simulink model "GDFLIB_FilterIIR1_BAM"  (Simulink 9.3)
settings: Solver=VariableStepAuto  StartTime=0.0  StopTime=10.0  RelTol=1e-3
settings Model: Creator=nxa18952  LastModifiedBy=nxa18952
settings DataIOCC: SaveFormat=Dataset  SignalLoggingSaveFormat=Dataset  ReturnWorkspaceOutputs=on
settings OptimizationCC: LifeSpan=auto
settings DebuggingCC: UnderspecifiedInitializationDetection=Simplified  MergeDetectMultiDrivingBlocksExec=error  FcnCallInpInsideContextMsg=error  SFUnexpectedBacktrackingDiag=error  SFNoUnconditionalDefaultTransitionDiag=error  SFExecutionAtInitializationDiag=warning  ArithmeticOperatorsInVariantConditions=error
settings HardwareCC: ProdBitPerPointer=64  ProdBitPerSizeT=64  ProdBitPerPtrDiffT=64  ProdLargestAtomicFloat=Float  ProdIntDivRoundTo=Zero  ProdEndianess=LittleEndian  ProdWordSize=64  ProdHWDeviceType=Intel->x86-64 (Windows64)
settings ModelReferenceCC: PropagateSignalLabelsOutOfModel=on
settings SFSimCC: SimUseLocalCustomCode=on
settings RTWCC: RTWUseLocalCustomCode=on
settings CodeAppCC: StateflowObjectComments=off
settings GRTTargetCC: TargetLangStandard=C99 (ISO)  CombineOutputUpdateFcns=on  GRTInterface=off
settings ConfigComp: CovMetricSettings=dwe  CovHtmlReporting=off  CovSaveCumulativeToWorkspaceVar=off  CovSaveSingleToWorkspaceVar=off  CovExternalEMLEnable=on

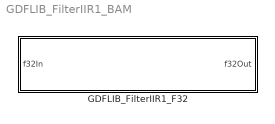
== system GDFLIB_FilterIIR1_BAM ==
  GDFLIB_FilterIIR1_F32 : Subsystem  TreatAsAtomicUnit=on  mask(GDFLIB_FilterIIR1_F32){showStates=Hide (faster execution), f32B0=0, f32B1=0, f32A1=0}
      mask prompts: showStates "Show internal states"; f32B0 "f32B0 (B0 coefficient of the IIR1 filter in 32-bit fixed-point fractional format)"; f32B1 "f32B1 (B1 coefficient of the IIR1 filter in 32-bit fixed-point fractional format)"; f32A1 "f32A1 (A1 coefficient of the IIR1 filter in 32-bit fixed-point fractional format)"
      mask help: Direct form I first order IIR filter in 32-bit fixed-point fractional implementation. Refer to the AMMCLIB User's Guide for further details.
      mask init:
      | if ~evalin('base','exist(''tS8'',''var'')')
      |   if (2 ~= exist('SWLIBS_Typedefs.mat','file'))
      |       error('File SWLIBS_Typedefs.mat is not on the Matlab path. Please add the AMMCLIB "bam" folder in the Matlab Search Path.');
      |   else
      |       evalin('base', 'load(''SWLIBS_Typedefs.mat'')');
      |   end
      | end
      | if showStates == 1
      |     % hidden state variables
      |     if strcmp(get_param([gcb '/f32B0'], 'BlockType'), 'Inport')
      |         posblk = get_param(gcb, 'Position');
      | 
      |         pos = get_param(    [gcb, '/f32B0'], 'Position');
      |         orient = get_param( [gcb, '/f32B0'], 'Orientation');
      |         delete_block(       [gcb, '/f32B0']);
      |         add_block('built-in/Ground', [gcb, '/f32B0'], 'Position', pos, 'Orientation', orient);
      | 
      |         pos = get_param(    [gcb, '/f32B1'], 'Position');
      |         orient = get_param( [gcb, '/f32B1'], 'Orientation');
      |         delete_block(       [gcb, '/f32B1']);
      |         add_block('built-in/Ground', [gcb, '/f32B1'], 'Position', pos, 'Orientation', orient);
      | 
      |         pos = get_param(    [gcb, '/f32A1'], 'Position');
      |         orient = get_param( [gcb, '/f32A1'], 'Orientation');
      |         delete_block(       [gcb, '/f32A1']);
      |         add_block('built-in/Ground', [gcb, '/f32A1'], 'Position', pos, 'Orientation', orient);
      | 
      |         pos = get_param(    [gcb, '/f32FiltBufferX'], 'Position');
      |         orient = get_param( [gcb, '/f32FiltBufferX'], 'Orientation');
      |         delete_block(       [gcb, '/f32FiltBufferX']);
      |         add_block('built-in/Ground', [gcb, '/f32FiltBufferX'], 'Position', pos, 'Orientation', orient);
      | 
      |         pos = get_param(    [gcb, '/f32FiltBufferY'], 'Position');
      |         orient = get_param( [gcb, '/f32FiltBufferY'], 'Orientation');
      |         delete_block(       [gcb, '/f32FiltBufferY']);
      |         add_block('built-in/Ground', [gcb, '/f32FiltBufferY'], 'Position', pos, 'Orientation', orient);
      | 
      | 
      |         pos = get_param(    [gcb '/f32FiltBufferX_Out'], 'Position');
      |         orient = get_param( [gcb '/f32FiltBufferX_Out'], 'Orientation');
      |         delete_block(       [gcb '/f32FiltBufferX_Out']);
      |         add_block('built-in/Terminator', [gcb '/f32FiltBufferX_Out'], 'Position', pos, 'Orientation', orient);
      | 
      |         pos = get_param(    [gcb '/f32FiltBufferY_Out'], 'Position');
      |         orient = get_param( [gcb '/f32FiltBufferY_Out'], 'Orientation');
      |         delete_block(       [gcb '/f32FiltBufferY_Out']);
      |         add_block('built-in/Terminator', [gcb '/f32FiltBufferY_Out'], 'Position', pos, 'Orientation', orient);
      | 
      | 
      |         set_param([gcb '/f32In'], 'Port', '1');
      | 
      |         set_param([gcb '/f32Out'], 'Port', '1');
      | 
      |         set_param(gcb,'MaskEnables',{'on','on','on','on'});
      | 
      |         if (posblk(4) - posblk(2)) > 50
      |           height = 50;
      |           set_param(gcb,'Position',[posblk(1), posblk(2), posblk(3), posblk(2)+height])
      |         end
      |     end
      | else
      |     % shown state variables
      |     if strcmp(get_param([gcb '/f32B0'], 'BlockType'), 'Ground')
      |         posblk = get_param(gcb, 'Position');
      | 
      |         pos = get_param(    [gcb, '/f32B0'], 'Position');
      |         orient = get_param( [gcb, '/f32B0'], 'Orientation');
      |         delete_block(       [gcb, '/f32B0']);
      |         add_block('built-in/Inport', [gcb, '/f32B0'], 'Position', pos, 'Orientation', orient, 'OutDataTypeStr', 'int32');
      | 
      |         pos = get_param(    [gcb, '/f32B1'], 'Position');
      |         orient = get_param( [gcb, '/f32B1'], 'Orientation');
      |         delete_block(       [gcb, '/f32B1']);
      |         add_block('built-in/Inport', [gcb, '/f32B1'], 'Position', pos, 'Orientation', orient, 'OutDataTypeStr', 'int32');
      | 
      |         pos = get_param(    [gcb, '/f32A1'], 'Position');
      |         orient = get_param( [gcb, '/f32A1'], 'Orientation');
      |         delete_block(       [gcb, '/f32A1']);
      |         add_block('built-in/Inport', [gcb, '/f32A1'], 'Position', pos, 'Orientation', orient, 'OutDataTypeStr', 'int32');
      | 
      |         pos = get_param(    [gcb, '/f32FiltBufferX'], 'Position');
      |         orient = get_param( [gcb, '/f32FiltBufferX'], 'Orientation');
      |         delete_block(       [gcb, '/f32FiltBufferX']);
      |         add_block('built-in/Inport', [gcb, '/f32FiltBufferX'], 'Position', pos, 'Orientation', orient, 'OutDataTypeStr', 'int32');
      | 
      |         pos = get_param(    [gcb, '/f32FiltBufferY'], 'Position');
      |         orient = get_param( [gcb, '/f32FiltBufferY'], 'Orientation');
      |         delete_block(       [gcb, '/f32FiltBufferY']);
      |         add_block('built-in/Inport', [gcb, '/f32FiltBufferY'], 'Position', pos, 'Orientation', orient, 'OutDataTypeStr', 'int32');
      | 
      | 
      |         pos = get_param(    [gcb '/f32FiltBufferX_Out'], 'Position');
      |         orient = get_param( [gcb '/f32FiltBufferX_Out'], 'Orientation');
      |         delete_block(       [gcb '/f32FiltBufferX_Out']);
      |         add_block('built-in/Outport', [gcb '/f32FiltBufferX_Out'], 'Position', pos, 'Orientation', orient);
      | 
      |         pos = get_param(    [gcb '/f32FiltBufferY_Out'], 'Position');
      |         orient = get_param( [gcb '/f32FiltBufferY_Out'], 'Orientation');
      |         delete_block(       [gcb '/f32FiltBufferY_Out']);
      |         add_block('built-in/Outport', [gcb '/f32FiltBufferY_Out'], 'Position', pos, 'Orientation', orient);
      | 
      | 
      |         set_param([gcb '/f32In'], 'Port', '1');
      |         set_param([gcb '/f32B0'], 'Port', '2');
      |         set_param([gcb '/f32B1'], 'Port', '3');
      |         set_param([gcb '/f32A1'], 'Port', '4');
      |         set_param([gcb '/f32FiltBufferX'], 'Port', '5');
      |         set_param([gcb '/f32FiltBufferY'], 'Port', '6');
      | 
      |         set_param([gcb '/f32Out'], 'Port', '1');
      |         set_param([gcb '/f32FiltBufferX_Out'], 'Port', '2');
      |         set_param([gcb '/f32FiltBufferY_Out'], 'Port', '3');
      | 
      |         set_param(gcb,'MaskEnables',{'on','off','off','off'});
      | 
      |         if (posblk(4) - posblk(2)) < 175
      |           height = 175;
      |           set_param(gcb,'Position',[posblk(1), posblk(2), posblk(3), posblk(2)+height])
      |         end
      |     end
      | end
      settings: RTWSystemCode=Inline
      mask TypeOptions showStates: Hide (faster execution) | Show (allows debugging; connect feedback loops manually)
      mask Callback showStates:
      | maskStr = get_param(gcb,'showStates');
      | if strcmp(maskStr,'Hide (faster execution)'),
      |     set_param(gcb,'MaskEnables',{'on','on','on','on'});
      | else
      |     set_param(gcb,'MaskEnables',{'on','off','off','off'});
      | end
      mask Display:
      | color('black');
      | pos = get_param(gcb, 'Position');
      | width = pos(3) - pos(1);
      | height = pos(4) - pos(2);
      | tX=width/2;
      | tY=height - 8;
      | color('black');
      | text(tX,tY, 'GDFLIB_FilterIIR1_F32', 'horizontalAlignment', 'center');
      | if showStates == 2
      |   color('red');
      |   text(tX,tY - 20, ['debugging mode' char(13) char(10) '(limited performance)'], 'horizontalAlignment', 'center');
      | end

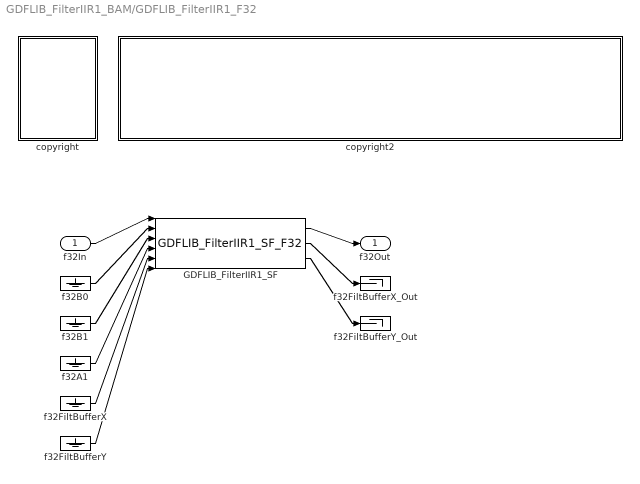
== system GDFLIB_FilterIIR1_BAM/GDFLIB_FilterIIR1_F32 ==
  f32In : Inport  OutDataTypeStr=int32
  GDFLIB_FilterIIR1_SF : S-Function  FunctionName=GDFLIB_FilterIIR1_SF_F32  Parameters=showStates,f32B0,f32B1,f32A1  SFunctionDeploymentMode=off  EnableBusSupport=off
  copyright : Subsystem
      mask Display: text(10,90,'FILE:');text(10,75,'DESRIPTION:');text(10,60,'COPYRIGHT:');text(10,45,'VERSION:');text(10,30,'DATE:')
  copyright2 : Subsystem
      mask Display: text(10,90,'GDFLIB_FilterIIR1_BAM_F32.mdl');text(10,75,'First order IIR filter.');text(10,60,'NXP 2020');text(10,45,'1.0');text(10,30,'18-Mar-2020');
  f32A1 : Ground
  f32B0 : Ground
  f32B1 : Ground
  f32FiltBufferX : Ground
  f32FiltBufferX_Out : Terminator
  f32FiltBufferY : Ground
  f32FiltBufferY_Out : Terminator
  f32Out : Outport
  wires:
  f32In/1 -> GDFLIB_FilterIIR1_SF/1
  f32B0/1 -> GDFLIB_FilterIIR1_SF/2
  f32B1/1 -> GDFLIB_FilterIIR1_SF/3
  f32A1/1 -> GDFLIB_FilterIIR1_SF/4
  f32FiltBufferX/1 -> GDFLIB_FilterIIR1_SF/5
  f32FiltBufferY/1 -> GDFLIB_FilterIIR1_SF/6
  GDFLIB_FilterIIR1_SF/1 -> f32Out/1
  GDFLIB_FilterIIR1_SF/2 -> f32FiltBufferX_Out/1
  GDFLIB_FilterIIR1_SF/3 -> f32FiltBufferY_Out/1

== system GDFLIB_FilterIIR1_BAM/GDFLIB_FilterIIR1_F32/copyright ==

== system GDFLIB_FilterIIR1_BAM/GDFLIB_FilterIIR1_F32/copyright2 ==
